simulink model "quadtanks_pid2"  (R2014b)
settings: Solver=ode45  StartTime=0.0  StopTime=10.0  RelTol=1e-3
values from neighbouring files (symbols this model uses):
  gs11_d = double(coeff_gs11(1))    [fase_minima.m]    (also in fase_nao_minima.m; model_minimum_phase.m; model_nonminimum_phase.m)
  gs11_ds = double(coeff_gs11(2))    [fase_minima.m]    (also in fase_nao_minima.m; model_minimum_phase.m; model_nonminimum_phase.m)
  gs11_n = gamma1*c1    [fase_minima.m]    (also in fase_nao_minima.m; model_minimum_phase.m; model_nonminimum_phase.m)
  gs12_d = double(coeff_gs12(1))    [fase_minima.m]    (also in fase_nao_minima.m; model_minimum_phase.m; model_nonminimum_phase.m)
  gs12_ds = double(coeff_gs12(2))    [fase_minima.m]    (also in fase_nao_minima.m; model_minimum_phase.m; model_nonminimum_phase.m)
  gs12_ds2 = double(coeff_gs12(3))    [fase_minima.m]    (also in fase_nao_minima.m; model_minimum_phase.m; model_nonminimum_phase.m)
  gs12_n = (1-gamma2)*c1    [fase_minima.m]    (also in fase_nao_minima.m; model_minimum_phase.m; model_nonminimum_phase.m)
  gs21_d = double(coeff_gs21(1))    [fase_minima.m]    (also in fase_nao_minima.m; model_minimum_phase.m; model_nonminimum_phase.m)
  gs21_ds = double(coeff_gs21(2))    [fase_minima.m]    (also in fase_nao_minima.m; model_minimum_phase.m; model_nonminimum_phase.m)
  gs21_ds2 = double(coeff_gs21(3))    [fase_minima.m]    (also in fase_nao_minima.m; model_minimum_phase.m; model_nonminimum_phase.m)
  gs21_n = (1-gamma1)*c2    [fase_minima.m]    (also in fase_nao_minima.m; model_minimum_phase.m; model_nonminimum_phase.m)
  gs22_d = double(coeff_gs22(1))    [fase_minima.m]    (also in fase_nao_minima.m; model_minimum_phase.m; model_nonminimum_phase.m)
  gs22_ds = double(coeff_gs22(2))    [fase_minima.m]    (also in fase_nao_minima.m; model_minimum_phase.m; model_nonminimum_phase.m)
  gs22_n = gamma2*c2    [fase_minima.m]    (also in fase_nao_minima.m; model_minimum_phase.m; model_nonminimum_phase.m)
  Kp1 = 0.78    [main.m]    (also in old_main.m)
  Kp2 = Kp1    (= 0.78)    [main.m]    (also in old_main.m)
  Td1 = 0    [main.m]    (also in old_main.m)
  Td2 = Td1    (= 0)    [main.m]    (also in old_main.m)
  Ti1 = 2.25    [main.m]    (also in old_main.m)
  Ti2 = Ti1    (= 2.25)    [main.m]    (also in old_main.m)
  W1 = eye(2)    [pid_minimum_phase.m]    (also in pid_nonminimum_phase.m)
  W2 = eye(2)    [pid_minimum_phase.m]    (also in pid_nonminimum_phase.m)
libraries: simulink x2
settings Model: Creator=cfppwin  LastModifiedBy=cfppwin

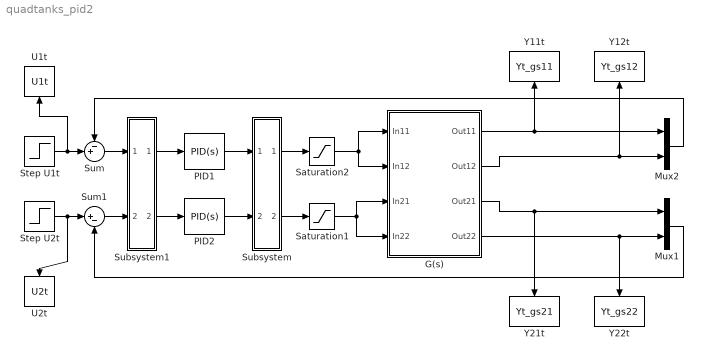
== system quadtanks_pid2 ==
  G(s) : Subsystem
  Mux1 : Mux  Inputs=2
  Mux2 : Mux  Inputs=2
  PID1 : simulink/Continuous/PID Controller  Controller=PID  TimeDomain=Continuous-time  SampleTime=-1  IntegratorMethod=Forward Euler  FilterMethod=Forward Euler  Form=Parallel  P=Kp1  I=Ti1  D=Td1  N=100  InitialConditionSource=internal  InitialConditionForIntegrator=0  InitialConditionForFilter=0  ExternalReset=none  LimitOutput=off  UpperSaturationLimit=inf  LowerSaturationLimit=-inf  LinearizeAsGain=on  AntiWindupMode=none  Kb=1  TrackingMode=off  Kt=1  PParamMin=[]  PParamMax=[]  IParamMin=[]  IParamMax=[]  DParamMin=[]  DParamMax=[]  NParamMin=[]  NParamMax=[]  KbParamMin=[]  KbParamMax=[]  KtParamMin=[]  KtParamMax=[]  POutMin=[]  POutMax=[]  IOutMin=[]  IOutMax=[]  DOutMin=[]  DOutMax=[]  NOutMin=[]  NOutMax=[]  KbOutMin=[]  KbOutMax=[]  KtOutMin=[]  KtOutMax=[]  IntegratorOutMin=[]  IntegratorOutMax=[]  FilterOutMin=[]  FilterOutMax=[]  SumOutMin=[]  SumOutMax=[]  SumI1OutMin=[]  SumI1OutMax=[]  SumI2OutMin=[]  SumI2OutMax=[]  SumI3OutMin=[]  SumI3OutMax=[]  SumDOutMin=[]  SumDOutMax=[]  SaturationOutMin=[]  SaturationOutMax=[]  IntegratorContinuousStateAttributes=''  IntegratorStateMustResolveToSignalObject=off  IntegratorRTWStateStorageClass=Auto  FilterContinuousStateAttributes=''  FilterStateMustResolveToSignalObject=off  FilterRTWStateStorageClass=Auto  DifferentiatorICPrevScaledInput=0  DifferentiatorOutMin=[]  DifferentiatorOutMax=[]  UseFilter=on
  PID2 : simulink/Continuous/PID Controller  Controller=PID  TimeDomain=Continuous-time  SampleTime=-1  IntegratorMethod=Forward Euler  FilterMethod=Forward Euler  Form=Parallel  P=Kp2  I=Ti2  D=Td2  N=100  InitialConditionSource=internal  InitialConditionForIntegrator=0  InitialConditionForFilter=0  ExternalReset=none  LimitOutput=off  UpperSaturationLimit=inf  LowerSaturationLimit=-inf  LinearizeAsGain=on  AntiWindupMode=none  Kb=1  TrackingMode=off  Kt=1  PParamMin=[]  PParamMax=[]  IParamMin=[]  IParamMax=[]  DParamMin=[]  DParamMax=[]  NParamMin=[]  NParamMax=[]  KbParamMin=[]  KbParamMax=[]  KtParamMin=[]  KtParamMax=[]  POutMin=[]  POutMax=[]  IOutMin=[]  IOutMax=[]  DOutMin=[]  DOutMax=[]  NOutMin=[]  NOutMax=[]  KbOutMin=[]  KbOutMax=[]  KtOutMin=[]  KtOutMax=[]  IntegratorOutMin=[]  IntegratorOutMax=[]  FilterOutMin=[]  FilterOutMax=[]  SumOutMin=[]  SumOutMax=[]  SumI1OutMin=[]  SumI1OutMax=[]  SumI2OutMin=[]  SumI2OutMax=[]  SumI3OutMin=[]  SumI3OutMax=[]  SumDOutMin=[]  SumDOutMax=[]  SaturationOutMin=[]  SaturationOutMax=[]  IntegratorContinuousStateAttributes=''  IntegratorStateMustResolveToSignalObject=off  IntegratorRTWStateStorageClass=Auto  FilterContinuousStateAttributes=''  FilterStateMustResolveToSignalObject=off  FilterRTWStateStorageClass=Auto  DifferentiatorICPrevScaledInput=0  DifferentiatorOutMin=[]  DifferentiatorOutMax=[]  UseFilter=on
  Saturation1 : Saturate  UpperLimit=10  LowerLimit=0
  Saturation2 : Saturate  UpperLimit=10  LowerLimit=0
  Step U1t : Step  Time=50  Before=5  After=6  SampleTime=0
  Step U2t : Step  Time=100  Before=5  After=6  SampleTime=0
  Subsystem : Subsystem
      mask Display: disp('W1')
  Subsystem1 : Subsystem
      mask Display: disp('W2')
  Sum : Sum  Inputs=-+|  SaturateOnIntegerOverflow=on  InputSameDT=on  OutDataTypeStr=Inherit: Same as first input
  Sum1 : Sum  Inputs=|+-  SaturateOnIntegerOverflow=on  InputSameDT=on  OutDataTypeStr=Inherit: Same as first input
  U1t : ToWorkspace  VariableName=U1t  SampleTime=-1
      settings: Save2DSignal=2-D array (concatenate along first dimension)
  U2t : ToWorkspace  VariableName=U2t  SampleTime=-1
      settings: Save2DSignal=2-D array (concatenate along first dimension)
  Y11t : ToWorkspace  VariableName=Yt_gs11  SampleTime=-1
      settings: Save2DSignal=2-D array (concatenate along first dimension)
  Y12t : ToWorkspace  VariableName=Yt_gs12  SampleTime=-1
      settings: Save2DSignal=2-D array (concatenate along first dimension)
  Y21t : ToWorkspace  VariableName=Yt_gs21  SampleTime=-1
      settings: Save2DSignal=2-D array (concatenate along first dimension)
  Y22t : ToWorkspace  VariableName=Yt_gs22  SampleTime=-1
      settings: Save2DSignal=2-D array (concatenate along first dimension)
  wires:
  Step U2t/1 -> U2t/1, Sum1/1
  PID1/1 -> Subsystem/1(In1)
  PID2/1 -> Subsystem/2(In2)
  Subsystem1/1(Out1) -> PID1/1
  Subsystem1/2(Out2) -> PID2/1
  Subsystem/1(Out1) -> Saturation2/1
  Subsystem/2(Out2) -> Saturation1/1
  Sum/1 -> Subsystem1/1(In1)
  Sum1/1 -> Subsystem1/2(In2)
  Step U1t/1 -> U1t/1, Sum/2
  Saturation2/1 -> G(s)/2(In12), G(s)/1(In11)
  Saturation1/1 -> G(s)/4(In22), G(s)/3(In21)
  G(s)/1(Out11) -> Y11t/1, Mux2/1
  G(s)/2(Out12) -> Y12t/1, Mux2/2
  G(s)/4(Out22) -> Y22t/1, Mux1/2
  G(s)/3(Out21) -> Y21t/1, Mux1/1
  Mux1/1 -> Sum1/2
  Mux2/1 -> Sum/1

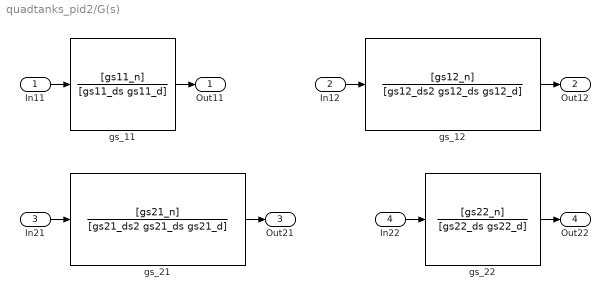
== system quadtanks_pid2/G(s) ==
  In11 : Inport
  In12 : Inport  Port=2
  In21 : Inport  Port=3
  In22 : Inport  Port=4
  gs_11 : TransferFcn  Numerator=[gs11_n]  Denominator=[gs11_ds gs11_d]
  gs_12 : TransferFcn  Numerator=[gs12_n]  Denominator=[gs12_ds2 gs12_ds gs12_d]
  "gs_21 " : TransferFcn  Numerator=[gs21_n]  Denominator=[gs21_ds2 gs21_ds gs21_d]
  gs_22 : TransferFcn  Numerator=[gs22_n]  Denominator=[gs22_ds gs22_d]
  Out11 : Outport
  Out12 : Outport  Port=2
  Out21 : Outport  Port=3
  Out22 : Outport  Port=4
  wires:
  "gs_21 "/1 -> Out21/1
  In12/1 -> gs_12/1
  gs_22/1 -> Out22/1
  In22/1 -> gs_22/1
  gs_11/1 -> Out11/1
  In11/1 -> gs_11/1
  In21/1 -> "gs_21 "/1
  gs_12/1 -> Out12/1

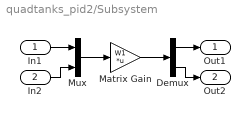
== system quadtanks_pid2/Subsystem ==
  In1 : Inport
  In2 : Inport  Port=2
  Demux : Demux  Outputs=2
  Matrix Gain : Gain  Gain=W1  Multiplication=Matrix(K*u)  SaturateOnIntegerOverflow=on  OutDataTypeStr=Inherit: Same as input  ParamDataTypeStr=Inherit: Same as input
  Mux : Mux  Inputs=2
  Out1 : Outport
  Out2 : Outport  Port=2
  wires:
  Demux/1 -> Out1/1
  In1/1 -> Mux/1
  Demux/2 -> Out2/1
  In2/1 -> Mux/2
  Mux/1 -> Matrix Gain/1
  Matrix Gain/1 -> Demux/1

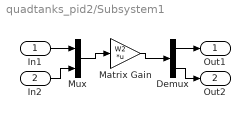
== system quadtanks_pid2/Subsystem1 ==
  In1 : Inport
  In2 : Inport  Port=2
  Demux : Demux  Outputs=2
  Matrix Gain : Gain  Gain=W2  Multiplication=Matrix(K*u)  SaturateOnIntegerOverflow=on  OutDataTypeStr=Inherit: Same as input  ParamDataTypeStr=Inherit: Same as input
  Mux : Mux  Inputs=2
  Out1 : Outport
  Out2 : Outport  Port=2
  wires:
  Matrix Gain/1 -> Demux/1
  Mux/1 -> Matrix Gain/1
  In2/1 -> Mux/2
  Demux/2 -> Out2/1
  In1/1 -> Mux/1
  Demux/1 -> Out1/1
